simulink model "UDPLink_Distal_wBoatIMU"  (R2020a)
settings: Solver=FixedStepAuto  StartTime=0.0  StopTime=inf  FixedStep=Ts  RelTol=1e-3  EnableMultiTasking=on
undefined symbols (not defined in the file or in its folder): IO392, standard
libraries: xpcutilitieslib x25, hdlsllib x15, slrtlib x4, simulink x3, speedgoatlib_fpga_quadrature x2, xpcrtudplib x2, xpcseriallib x1, speedgoatlib_fpga x1, speedgoatlib_IO581 x1
settings Model: SimulationMode=external  Creator=ViconLab  LastModifiedBy=mae-vermillionlab
settings SolverCC: ConcurrentTasks=on  AutoInsertRateTranBlk=on
settings DataIOCC: SaveFormat=StructureWithTime
settings OptimizationCC: BlockReduction=off  OptimizeBlockIOStorage=off
settings HardwareCC: ProdBitPerPointer=32  ProdBitPerSizeT=32  ProdBitPerPtrDiffT=32  ProdLargestAtomicFloat=None  ProdWordSize=32  ProdLongLongMode=on  ProdHWDeviceType=Generic->32-bit x86 compatible
settings RTWCC: Description=Simulink Real-Time  SystemTargetFile=slrt.tlc  TemplateMakefile=slrt_default_tmf  CodeExecutionProfiling=on  RTWCompilerOptimization=on
settings SimulinkRealTimeCC: SupportVariableSizeSignals=on  RL32LogTETModifier=off  xPCConcurrentTasks=on

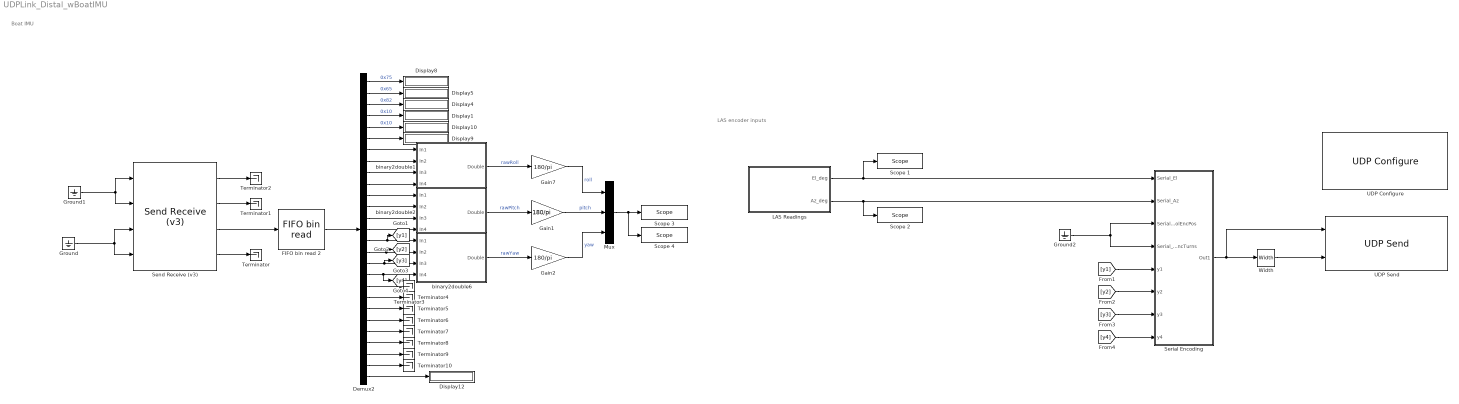
== system UDPLink_Distal_wBoatIMU ==
  note: Boat IMU
  note: LAS encoder inputs
  Demux2 : Demux  Outputs=27
  Display{1,4..5,8..10,12} (7 alike) : Display
      settings: Format=hex (Stored Integer)
  FIFO bin read 2 : xpcseriallib/FIFO bin read   header={[0x75 0x65 0x82 0x10]}  lengths=[26]  hold=Hold last output if no new data  enable=off  maxsize=26  outputtype=8 bit uint null terminated  sampletime=0.01
      settings: SourceProductBaseCode=XP
  Gain1 : Gain  Gain=180/pi
  Gain2 : Gain  Gain=180/pi
  Gain7 : Gain  Gain=180/pi
  Ground : Ground
  Ground1 : Ground
  Ground2 : Ground
  "LAS Readings " : Subsystem
  Mux : Mux  Inputs=3
  Scope 1 : slrtlib/Displays and Logging/Scope   scopeno=1  scopetype=Target  autostart=on  viewmode=Graphical sliding  formatstr='%15.6f'  grid=on  ylimits=[0,8000]  nosamples=500  noprepostsamples=0  interleave=1  triggermode=FreeRun  triggersignal=1  trigsignalfromport=off  triggerlevel=0.0  triggerslope=Either  triggerscope=1  triggersample=0  filename=data.dat  mode=Lazy  writesize=512  autorestart=off  dynamicfilemode=off  maxwritefilesize=512*1024^2
  Scope 2 : slrtlib/Displays and Logging/Scope   scopeno=2  scopetype=Target  autostart=on  viewmode=Graphical sliding  formatstr='%15.6f'  grid=on  ylimits=[0,8000]  nosamples=500  noprepostsamples=0  interleave=1  triggermode=FreeRun  triggersignal=1  trigsignalfromport=off  triggerlevel=0.0  triggerslope=Either  triggerscope=1  triggersample=0  filename=data.dat  mode=Lazy  writesize=512  autorestart=off  dynamicfilemode=off  maxwritefilesize=512*1024^2
  Scope 3 : slrtlib/Displays and Logging/Scope   scopeno=3  scopetype=Target  autostart=on  viewmode=Graphical sliding  formatstr='%15.6f'  grid=on  ylimits=[-180,180]  nosamples=250  noprepostsamples=0  interleave=1  triggermode=FreeRun  triggersignal=1  trigsignalfromport=off  triggerlevel=0.0  triggerslope=Either  triggerscope=1  triggersample=0  filename=data.dat  mode=Lazy  writesize=512  autorestart=off  dynamicfilemode=off  maxwritefilesize=512*1024^2
  Scope 4 : slrtlib/Displays and Logging/Scope   scopeno=4  scopetype=Target  autostart=on  viewmode=Numerical  formatstr='%15.6f'  grid=on  ylimits=[-180,180]  nosamples=250  noprepostsamples=0  interleave=1  triggermode=FreeRun  triggersignal=1  trigsignalfromport=off  triggerlevel=0.0  triggerslope=Either  triggerscope=1  triggersample=0  filename=data.dat  mode=Lazy  writesize=512  autorestart=off  dynamicfilemode=off  maxwritefilesize=512*1024^2
  "Send Receive (v3) " : speedgoatlib_IO581/Send Receive (v3)   parModuleId=1  parSlot=-1  parModuleType=IO581  parTransceiver12=RS485 Half-Duplex  parTransceiver34=RS232  parTransceiver1=RS485 Half-Duplex  parAutoTurnaround1=off  parTurnaroundDelay1=0  parStandardBaud1=on  parBaudrate1=115200  parBaudDivisor1=1  parSamplingRate1=16x (standard)  parPrescale1=off  parCalcBaud1=7812500  parParity1=None  parDataBits1=8  parStopBits1=1  parTxTrigLvl1=1  parRxTrigLvl1=1  parHandshake1=none  parRtsHysteresis1=0  parXon1=17  parXoff1=19  parTxSwFifoSize1=1024  parTxSwFifoType1=8 bit uint null terminated  parRxSwFifoSize1=1024  parTransceiver2=RS485 Half-Duplex  parAutoTurnaround2=off  parTurnaroundDelay2=0  parStandardBaud2=on  parBaudrate2=115200  parBaudDivisor2=1  parSamplingRate2=16x (standard)  parPrescale2=off  parCalcBaud2=7812500  parParity2=None  parDataBits2=8  parStopBits2=1  parTxTrigLvl2=1  parRxTrigLvl2=1  parHandshake2=none  parRtsHysteresis2=0  parXon2=17  parXoff2=19  parTxSwFifoSize2=1024  parTxSwFifoType2=8 bit uint null terminated  parRxSwFifoSize2=1024  parTransceiver3=RS232  parAutoTurnaround3=off  parTurnaroundDelay3=0  parStandardBaud3=on  parBaudrate3=115200  parBaudDivisor3=1  parSamplingRate3=16x (standard)  parPrescale3=off  parCalcBaud3=7812500  parParity3=None  parDataBits3=8  parStopBits3=1  parTxTrigLvl3=1  parRxTrigLvl3=8  parHandshake3=none  parRtsHysteresis3=0  parXon3=17  parXoff3=19  parTxSwFifoSize3=1024  parTxSwFifoType3=8 bit uint null terminated  parRxSwFifoSize3=1024  parTransceiver4=RS232  parAutoTurnaround4=off  parTurnaroundDelay4=0  parStandardBaud4=on  parBaudrate4=115200  parBaudDivisor4=1  parSamplingRate4=16x (standard)  parPrescale4=off  parCalcBaud4=7812500  parParity4=None  parDataBits4=8  parStopBits4=1  parTxTrigLvl4=1  parRxTrigLvl4=1  parHandshake4=none  parRtsHysteresis4=0  parXon4=17  parXoff4=19  parTxSwFifoSize4=1024  parTxSwFifoType4=8 bit uint null terminated  parRxSwFifoSize4=1024
      settings: SourceProductName=Simulink Real-Time: Speedgoat Library
  Serial Encoding : Subsystem
  Terminator{,1..10} (11 alike) : Terminator
  UDP Configure : xpcrtudplib/UDP Configure  Priority=-1  IpAddress=30.30.30.2  SubnetMask=255.255.255.0  Gateway=0.0.0.0  PciBus=13  PciSlot=0  PciFunction=0  ID=1  tune=0  disable=off  enableMulticast=off  MulticastIpAddress={}  MulticastMask={}
      settings: SourceProductBaseCode=XP
  UDP Send : xpcrtudplib/UDP Send  ipAddressVal=30.30.30.2  localPort=-1  toAddress=30.30.30.1  toPort=25001  sampleTime=Ts
      settings: SourceProductBaseCode=XP
  Width : Width
  binary2double1 : Subsystem
  binary2double2 : Subsystem
  binary2double6 : Subsystem
  wires:
  "LAS Readings "/1(El_deg) -> Serial Encoding/1("Serial_El "), Scope 1/1
  "LAS Readings "/2(Az_deg) -> Serial Encoding/2(Serial_Az), Scope 2/1
  Width/1 -> UDP Send/2
  Serial Encoding/1(Out1) -> UDP Send/1, Width/1
  Demux2/3 -> Display4/1  "0x82"
  "Send Receive (v3) "/3 -> FIFO bin read 2/1
  "Send Receive (v3) "/2 -> Terminator1/1
  FIFO bin read 2/1 -> Demux2/1
  Demux2/24 -> Terminator8/1
  Ground1/1 -> "Send Receive (v3) "/1, "Send Receive (v3) "/2
  Demux2/4 -> Display1/1  "0x10"
  "Send Receive (v3) "/4 -> Terminator/1
  Demux2/8 -> binary2double1/2(In2)
  Ground/1 -> "Send Receive (v3) "/4, "Send Receive (v3) "/3
  Demux2/16 -> [y2], binary2double6/2(In2)
  Demux2/15 -> [y1], binary2double6/1(In1)
  Demux2/7 -> binary2double1/1(In1)
  Demux2/10 -> binary2double1/4(In4)
  Demux2/23 -> Terminator7/1
  Demux2/2 -> Display5/1  "0x65"
  Demux2/14 -> binary2double2/4(In4)
  Demux2/5 -> Display10/1  "0x10"
  Demux2/19 -> Terminator3/1
  Demux2/26 -> Terminator10/1
  Demux2/25 -> Terminator9/1
  Demux2/13 -> binary2double2/3(In3)
  Demux2/1 -> Display8/1  "0x75"
  binary2double2/1(Double) -> Gain1/1  "rawPitch"
  Demux2/12 -> binary2double2/2(In2)
  "Send Receive (v3) "/1 -> Terminator2/1
  Demux2/11 -> binary2double2/1(In1)
  Demux2/18 -> [y4], binary2double6/4(In4)
  Demux2/17 -> [y3], binary2double6/3(In3)
  binary2double6/1(Double) -> Gain2/1  "rawYaw"
  Demux2/22 -> Terminator6/1
  Demux2/9 -> binary2double1/3(In3)
  binary2double1/1(Double) -> Gain7/1  "rawRoll"
  Demux2/6 -> Display9/1
  Demux2/20 -> Terminator4/1
  Demux2/21 -> Terminator5/1
  Demux2/27 -> Display12/1
  Gain2/1 -> Mux/3  "yaw"
  Gain1/1 -> Mux/2  "pitch"
  Gain7/1 -> Mux/1  "roll"
  Mux/1 -> Scope 4/1, Scope 3/1
  [y1] -> Serial Encoding/5(y1)
  [y2] -> Serial Encoding/6(y2)
  [y3] -> Serial Encoding/7(y3)
  [y4] -> Serial Encoding/8(y4)
  Ground2/1 -> Serial Encoding/4(Serial_SpoolEncTurns), Serial Encoding/3(Serial_SpoolEncPos)

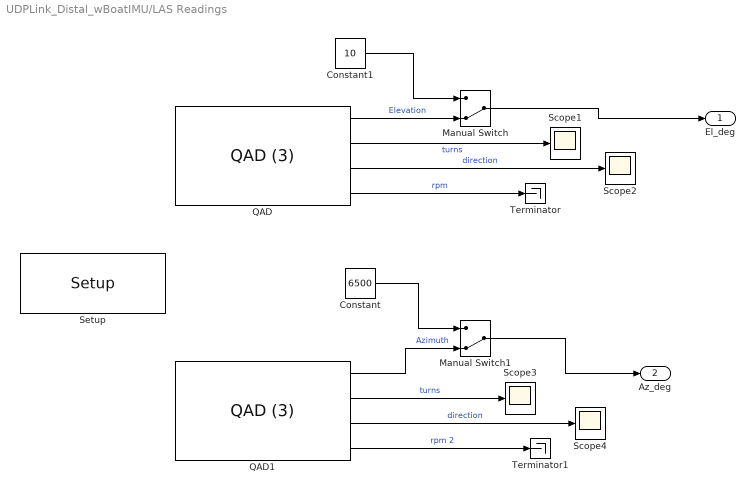
== system UDPLink_Distal_wBoatIMU/LAS Readings  ==
  Constant : Constant  Value=6500
  Constant1 : Constant  Value=10
  Manual Switch : ManualSwitch  CurrentSetting=0
  Manual Switch1 : ManualSwitch  CurrentSetting=0
  QAD : speedgoatlib_fpga_quadrature/QAD (3)  id=1  board=IO392-50k  chan=[2]  resetOnStart=on  ts=Ts  pciSlot=-1  operatingMode=Quadrature decoder  indexControlMode=Reset on index  resolution=4x  stepsPerRevolution=[8191]  latchMode=Disabled  interpolatePosition=off  invertAB=off  showClearPositionInput=off  showClearIndexFoundInput=off  showPositionOutput=on  showTurnOutput=on  showSpeedOutput=on  showDirectionOutput=on  showIndexFoundOutput=off
      settings: SourceProductName=Simulink Real-Time: Speedgoat I/O Driver Library
  QAD1 : speedgoatlib_fpga_quadrature/QAD (3)  id=1  board=IO392-50k  chan=[1]  resetOnStart=on  ts=Ts  pciSlot=-1  operatingMode=Quadrature decoder  indexControlMode=Reset on index  resolution=4x  stepsPerRevolution=[8191]  latchMode=Disabled  interpolatePosition=off  invertAB=off  showClearPositionInput=off  showClearIndexFoundInput=off  showPositionOutput=on  showTurnOutput=on  showSpeedOutput=on  showDirectionOutput=on  showIndexFoundOutput=off
      settings: SourceProductName=Simulink Real-Time: Speedgoat I/O Driver Library
  Scope{1..4} (4 alike) : Scope
  Setup : speedgoatlib_fpga/Setup/Setup  board=IO392-50k  id=1  device_id=1  frontIO=None  rearIO=None  bitstreamFile=speedgoat_IO392_50k_CI_02244.mat  rev=1.0  timestamp_string=07/12/20 12:10:05  fpgaFreq=75 MHz  fpgaTick=13.33 ns  ProgSpiFlash=off  ProgBPIFlash=off  pciSlot=-1  PullRPort0=pull-up 3.3V  VioPort0=3.3V  PullRPort1=pull-up 3.3V  VioPort1=3.3V  PullRPort2=pull-up 3.3V  VioPort2=3.3V  PullRPort3=pull-up 3.3V  VioPort3=3.3V  PullRPort4=pull-up 3.3V  VioPort4=3.3V  PullRPort5=pull-up 3.3V  VioPort5=3.3V  PullRPort6=pull-up 3.3V  VioPort6=3.3V  PullRPort15=pull-up 3.3V  PullRPort31=pull-up 3.3V  PullRPort47=pull-up 3.3V  PullRPort63=pull-up 3.3V
      settings: SourceProductName=Simulink Real-Time: Speedgoat Library
  Terminator : Terminator
  Terminator1 : Terminator
  El_deg : Outport
  Az_deg : Outport  Port=2
  wires:
  QAD1/2 -> Scope3/1  "turns"
  QAD/3 -> Scope2/1  "direction"
  QAD/4 -> Terminator/1  "rpm"
  QAD1/3 -> Scope4/1  "direction"
  QAD/2 -> Scope1/1  "turns"
  QAD1/4 -> Terminator1/1  "rpm 2"
  QAD/1 -> Manual Switch/2  "Elevation"
  Manual Switch/1 -> El_deg/1
  QAD1/1 -> Manual Switch1/2  "Azimuth"
  Manual Switch1/1 -> Az_deg/1
  Constant/1 -> Manual Switch1/1
  Constant1/1 -> Manual Switch/1

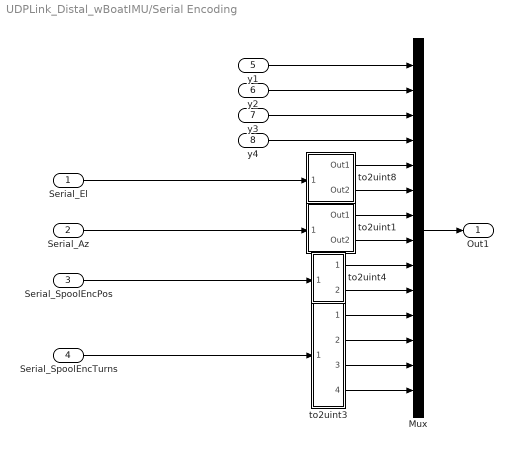
== system UDPLink_Distal_wBoatIMU/Serial Encoding ==
  "Serial_El " : Inport
  Serial_Az : Inport  Port=2
  Serial_SpoolEncPos : Inport  Port=3
  Serial_SpoolEncTurns : Inport  Port=4
  y1 : Inport  Port=5
  y2 : Inport  Port=6
  y3 : Inport  Port=7
  y4 : Inport  Port=8
  Mux : Mux  Inputs=14
  to2uint1 : Subsystem
  to2uint3 : Subsystem
  to2uint4 : Subsystem
  to2uint8 : Subsystem
  Out1 : Outport
  wires:
  "Serial_El "/1 -> to2uint8/1(" ")
  Serial_Az/1 -> to2uint1/1(" ")
  y3/1 -> Mux/3
  y4/1 -> Mux/4
  to2uint8/1(Out1) -> Mux/5
  to2uint8/2(Out2) -> Mux/6
  to2uint1/1(Out1) -> Mux/7
  to2uint1/2(Out2) -> Mux/8
  Mux/1 -> Out1/1
  y2/1 -> Mux/2
  y1/1 -> Mux/1
  to2uint3/1(Out4) -> Mux/11
  to2uint3/2(Out3) -> Mux/12
  to2uint3/3(Out1) -> Mux/13
  to2uint3/4(Out2) -> Mux/14
  Serial_SpoolEncTurns/1 -> to2uint3/1(" ")
  to2uint4/1(Out1) -> Mux/9
  to2uint4/2(Out2) -> Mux/10
  Serial_SpoolEncPos/1 -> to2uint4/1(" ")

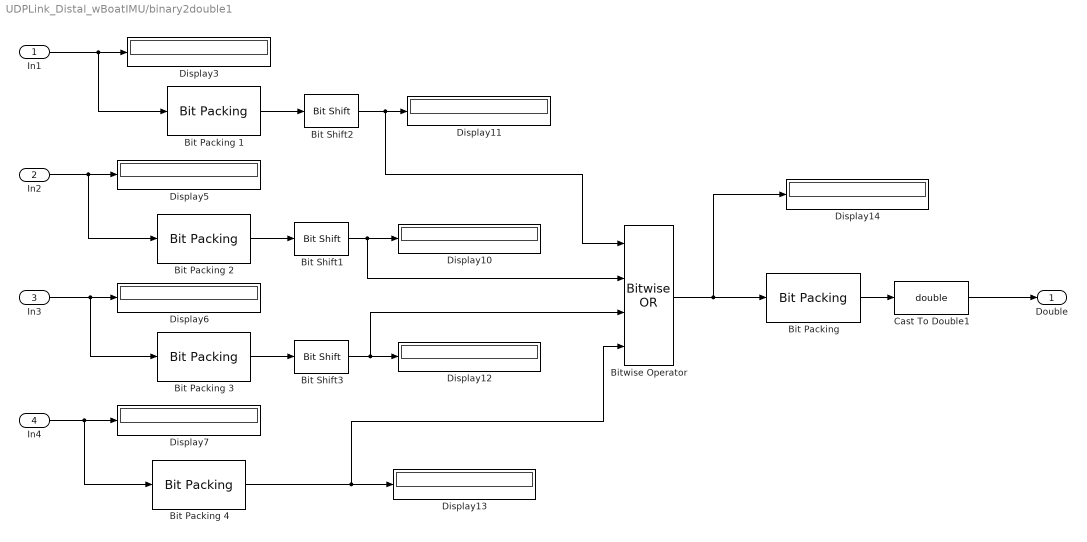
== system UDPLink_Distal_wBoatIMU/binary2double1 ==
  In1 : Inport
  In2 : Inport  Port=2
  In3 : Inport  Port=3
  In4 : Inport  Port=4
  Bit Packing {,1..4} (5 alike) : xpcutilitieslib/Bit Packing 
      settings: SourceProductBaseCode=XP
  Bit Shift1 : hdlsllib/Logic and Bit Operations/Bit Shift  mode=Shift Left Logical  N=16
  Bit Shift2 : hdlsllib/Logic and Bit Operations/Bit Shift  mode=Shift Left Logical  N=24
  Bit Shift3 : hdlsllib/Logic and Bit Operations/Bit Shift  mode=Shift Left Logical  N=8
  Bitwise Operator : simulink/Logic and Bit Operations/Bitwise Operator  logicop=OR  UseBitMask=off  NumInputPorts=4  BitMask=bin2dec('00000000')  BitMaskRealWorld=Stored Integer
  Cast To Double1 : DataTypeConversion  OutDataTypeStr=double
  Display{3,5..7,10..14} (9 alike) : Display
      settings: Format=hex (Stored Integer)
  Double : Outport
  wires:
  Bit Shift1/1 -> Bitwise Operator/2, Display10/1
  Bitwise Operator/1 -> Display14/1, "Bit Packing "/1
  Bit Packing 1/1 -> Bit Shift2/1
  Bit Packing 4/1 -> Bitwise Operator/4, Display13/1
  In1/1 -> Bit Packing 1/1, Display3/1
  In3/1 -> Bit Packing 3/1, Display6/1
  Bit Shift2/1 -> Bitwise Operator/1, Display11/1
  Bit Packing 2/1 -> Bit Shift1/1
  "Bit Packing "/1 -> Cast To Double1/1
  Bit Shift3/1 -> Bitwise Operator/3, Display12/1
  Bit Packing 3/1 -> Bit Shift3/1
  In2/1 -> Bit Packing 2/1, Display5/1
  In4/1 -> Bit Packing 4/1, Display7/1
  Cast To Double1/1 -> Double/1

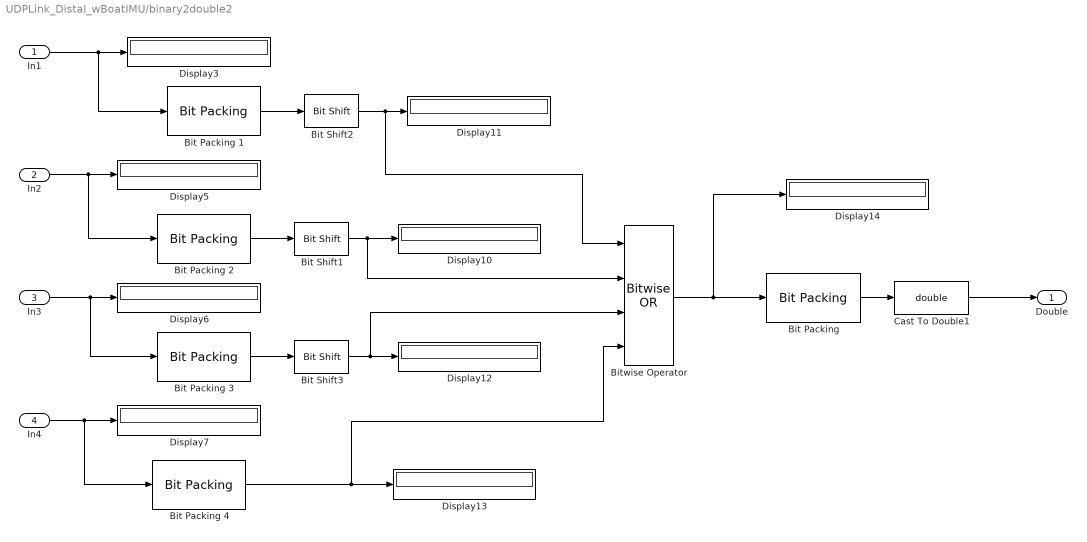
== system UDPLink_Distal_wBoatIMU/binary2double2 ==
  In1 : Inport
  In2 : Inport  Port=2
  In3 : Inport  Port=3
  In4 : Inport  Port=4
  Bit Packing {,1..4} (5 alike) : xpcutilitieslib/Bit Packing 
      settings: SourceProductBaseCode=XP
  Bit Shift1 : hdlsllib/Logic and Bit Operations/Bit Shift  mode=Shift Left Logical  N=16
  Bit Shift2 : hdlsllib/Logic and Bit Operations/Bit Shift  mode=Shift Left Logical  N=24
  Bit Shift3 : hdlsllib/Logic and Bit Operations/Bit Shift  mode=Shift Left Logical  N=8
  Bitwise Operator : simulink/Logic and Bit Operations/Bitwise Operator  logicop=OR  UseBitMask=off  NumInputPorts=4  BitMask=bin2dec('00000000')  BitMaskRealWorld=Stored Integer
  Cast To Double1 : DataTypeConversion  OutDataTypeStr=double
  Display{3,5..7,10..14} (9 alike) : Display
      settings: Format=hex (Stored Integer)
  Double : Outport
  wires:
  Cast To Double1/1 -> Double/1
  In4/1 -> Display7/1, Bit Packing 4/1
  In2/1 -> Display5/1, Bit Packing 2/1
  Bit Packing 3/1 -> Bit Shift3/1
  Bit Shift3/1 -> Display12/1, Bitwise Operator/3
  "Bit Packing "/1 -> Cast To Double1/1
  Bit Packing 2/1 -> Bit Shift1/1
  Bit Shift2/1 -> Display11/1, Bitwise Operator/1
  In3/1 -> Display6/1, Bit Packing 3/1
  In1/1 -> Display3/1, Bit Packing 1/1
  Bit Packing 4/1 -> Display13/1, Bitwise Operator/4
  Bit Packing 1/1 -> Bit Shift2/1
  Bitwise Operator/1 -> "Bit Packing "/1, Display14/1
  Bit Shift1/1 -> Display10/1, Bitwise Operator/2

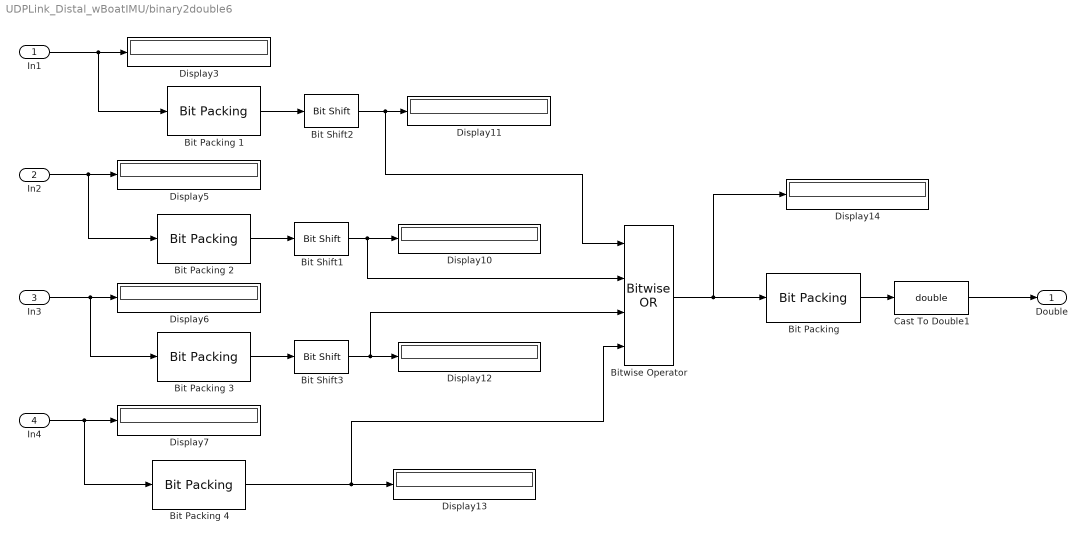
== system UDPLink_Distal_wBoatIMU/binary2double6 ==
  In1 : Inport
  In2 : Inport  Port=2
  In3 : Inport  Port=3
  In4 : Inport  Port=4
  Bit Packing {,1..4} (5 alike) : xpcutilitieslib/Bit Packing 
      settings: SourceProductBaseCode=XP
  Bit Shift1 : hdlsllib/Logic and Bit Operations/Bit Shift  mode=Shift Left Logical  N=16
  Bit Shift2 : hdlsllib/Logic and Bit Operations/Bit Shift  mode=Shift Left Logical  N=24
  Bit Shift3 : hdlsllib/Logic and Bit Operations/Bit Shift  mode=Shift Left Logical  N=8
  Bitwise Operator : simulink/Logic and Bit Operations/Bitwise Operator  logicop=OR  UseBitMask=off  NumInputPorts=4  BitMask=bin2dec('00000000')  BitMaskRealWorld=Stored Integer
  Cast To Double1 : DataTypeConversion  OutDataTypeStr=double
  Display{3,5..7,10..14} (9 alike) : Display
      settings: Format=hex (Stored Integer)
  Double : Outport
  wires:
  Bit Shift1/1 -> Bitwise Operator/2, Display10/1
  Bitwise Operator/1 -> Display14/1, "Bit Packing "/1
  Bit Packing 1/1 -> Bit Shift2/1
  Bit Packing 4/1 -> Bitwise Operator/4, Display13/1
  In1/1 -> Bit Packing 1/1, Display3/1
  In3/1 -> Bit Packing 3/1, Display6/1
  Bit Shift2/1 -> Bitwise Operator/1, Display11/1
  Bit Packing 2/1 -> Bit Shift1/1
  "Bit Packing "/1 -> Cast To Double1/1
  Bit Shift3/1 -> Bitwise Operator/3, Display12/1
  Bit Packing 3/1 -> Bit Shift3/1
  In2/1 -> Bit Packing 2/1, Display5/1
  In4/1 -> Bit Packing 4/1, Display7/1
  Cast To Double1/1 -> Double/1

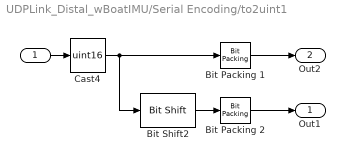
== system UDPLink_Distal_wBoatIMU/Serial Encoding/to2uint1 ==
  " " : Inport
  Bit Packing 1 : xpcutilitieslib/Bit Packing   MaskBitPatterns={[0:7]}  MaskPackDataType=uint8  MaskPackDataSize=[1]
      settings: SourceProductBaseCode=XP
  Bit Packing 2 : xpcutilitieslib/Bit Packing   MaskBitPatterns={[0:7]}  MaskPackDataType=uint8  MaskPackDataSize=[1]
      settings: SourceProductBaseCode=XP
  Bit Shift2 : hdlsllib/Logic and Bit Operations/Bit Shift  mode=Shift Right Arithmetic  N=8
  Cast4 : DataTypeConversion  OutDataTypeStr=uint16
  Out1 : Outport
  Out2 : Outport  Port=2
  wires:
  " "/1 -> Cast4/1
  Cast4/1 -> Bit Packing 1/1, Bit Shift2/1
  Bit Shift2/1 -> Bit Packing 2/1
  Bit Packing 2/1 -> Out1/1
  Bit Packing 1/1 -> Out2/1

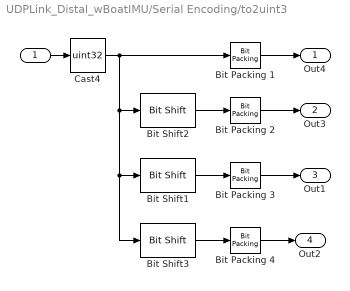
== system UDPLink_Distal_wBoatIMU/Serial Encoding/to2uint3 ==
  " " : Inport
  Bit Packing {1..4} (4 alike) : xpcutilitieslib/Bit Packing   MaskBitPatterns={[0:7]}  MaskPackDataType=uint8  MaskPackDataSize=[1]
      settings: SourceProductBaseCode=XP
  Bit Shift1 : hdlsllib/Logic and Bit Operations/Bit Shift  mode=Shift Right Arithmetic  N=16
  Bit Shift2 : hdlsllib/Logic and Bit Operations/Bit Shift  mode=Shift Right Arithmetic  N=8
  Bit Shift3 : hdlsllib/Logic and Bit Operations/Bit Shift  mode=Shift Right Arithmetic  N=24
  Cast4 : DataTypeConversion  OutDataTypeStr=uint32
  Out4 : Outport
  Out3 : Outport  Port=2
  Out1 : Outport  Port=3
  Out2 : Outport  Port=4
  wires:
  Bit Shift3/1 -> Bit Packing 4/1
  Bit Shift1/1 -> Bit Packing 3/1
  Bit Shift2/1 -> Bit Packing 2/1
  Cast4/1 -> Bit Shift2/1, Bit Shift3/1, Bit Shift1/1, Bit Packing 1/1
  " "/1 -> Cast4/1
  Bit Packing 3/1 -> Out1/1
  Bit Packing 4/1 -> Out2/1
  Bit Packing 2/1 -> Out3/1
  Bit Packing 1/1 -> Out4/1

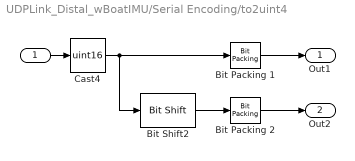
== system UDPLink_Distal_wBoatIMU/Serial Encoding/to2uint4 ==
  " " : Inport
  Bit Packing 1 : xpcutilitieslib/Bit Packing   MaskBitPatterns={[0:7]}  MaskPackDataType=uint8  MaskPackDataSize=[1]
      settings: SourceProductBaseCode=XP
  Bit Packing 2 : xpcutilitieslib/Bit Packing   MaskBitPatterns={[0:7]}  MaskPackDataType=uint8  MaskPackDataSize=[1]
      settings: SourceProductBaseCode=XP
  Bit Shift2 : hdlsllib/Logic and Bit Operations/Bit Shift  mode=Shift Right Arithmetic  N=8
  Cast4 : DataTypeConversion  OutDataTypeStr=uint16
  Out1 : Outport
  Out2 : Outport  Port=2
  wires:
  " "/1 -> Cast4/1
  Cast4/1 -> Bit Packing 1/1, Bit Shift2/1
  Bit Shift2/1 -> Bit Packing 2/1
  Bit Packing 1/1 -> Out1/1
  Bit Packing 2/1 -> Out2/1

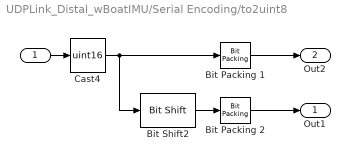
== system UDPLink_Distal_wBoatIMU/Serial Encoding/to2uint8 ==
  " " : Inport
  Bit Packing 1 : xpcutilitieslib/Bit Packing   MaskBitPatterns={[0:7]}  MaskPackDataType=uint8  MaskPackDataSize=[1]
      settings: SourceProductBaseCode=XP
  Bit Packing 2 : xpcutilitieslib/Bit Packing   MaskBitPatterns={[0:7]}  MaskPackDataType=uint8  MaskPackDataSize=[1]
      settings: SourceProductBaseCode=XP
  Bit Shift2 : hdlsllib/Logic and Bit Operations/Bit Shift  mode=Shift Right Arithmetic  N=8
  Cast4 : DataTypeConversion  OutDataTypeStr=uint16
  Out1 : Outport
  Out2 : Outport  Port=2
  wires:
  Bit Shift2/1 -> Bit Packing 2/1
  Cast4/1 -> Bit Shift2/1, Bit Packing 1/1
  " "/1 -> Cast4/1
  Bit Packing 2/1 -> Out1/1
  Bit Packing 1/1 -> Out2/1
